simulink model "Invented_system_simulink_try"  (R2018b)
settings: Solver=VariableStepAuto  StartTime=0.0  StopTime=50  MaxStep=0.01  MinStep=0.00005  RelTol=1e-3
settings Model: Creator=ahmed  LastModifiedBy=ahmed

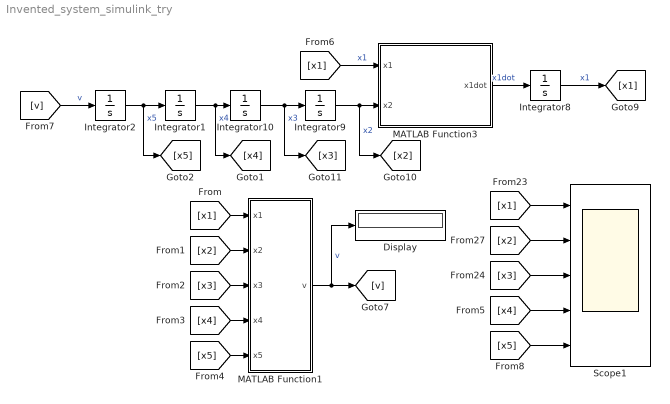
== system Invented_system_simulink_try ==
  Display : Display
      settings: Decimation=3
  Integrator1 : Integrator  InitialCondition=10
  Integrator10 : Integrator  InitialCondition=10
  Integrator2 : Integrator  InitialCondition=10
  Integrator8 : Integrator  InitialCondition=-10
  Integrator9 : Integrator  InitialCondition=20
  MATLAB Function1 : MATLAB Function  TreatAsAtomicUnit=on
  MATLAB Function3 : MATLAB Function  TreatAsAtomicUnit=on
  Scope1 : Scope  NumInputPorts=5
  wires:
  [x2] -> MATLAB Function1/2(x2)
  MATLAB Function1/1(v) -> Display/1, [v]  "v"
  [x1] -> Scope1/1
  [x1] -> MATLAB Function1/1(x1)
  [x3] -> MATLAB Function1/3(x3)
  MATLAB Function3/1(x1dot) -> Integrator8/1  "x1dot"
  Integrator8/1 -> [x1]  "x1"
  [x1] -> MATLAB Function3/1(x1)  "x1"
  Integrator9/1 -> [x2], MATLAB Function3/2(x2)  "x2"
  Integrator10/1 -> [x3], Integrator9/1  "x3"
  [v] -> Integrator2/1  "v"
  [x3] -> Scope1/3
  [x2] -> Scope1/2
  Integrator1/1 -> [x4], Integrator10/1  "x4"
  Integrator2/1 -> [x5], Integrator1/1  "x5"
  [x4] -> MATLAB Function1/4(x4)
  [x5] -> MATLAB Function1/5(x5)
  [x4] -> Scope1/4
  [x5] -> Scope1/5

== matlab function Invented_system_simulink_try/MATLAB Function1 ==
  data: x1 input; v output; x2 input; x3 input; x4 input; x5 input
function v = fcn(x1,x2,x3,x4,x5)

% Max step size 0.01
% Min step size auto
% not working initial conditions: x1=-10, x2=20, x3=10, x4=10, x5=10
% working initial conditions: x1=-10, x2=20, x3=-10, x4=10, x5=-10
% working initial conditions: x1=10, x2=20, x3=30, x4=40, x5=50
% working initial conditions: x1=1, x2=2, x3=3, x4=4, x5=5

% Max step size 0.01
% Min step size 0.00005
% all working

e2 = x2 + x1 + cos(x1);
e3 = x3 + 2*e2 - e2*sin(x1) + x1*sin(x1);

e4 = x4 + 3*e3 - e2 - 2*x1 - e3*sin(x1) + 2*e2*sin(x1) - e2^2*cos(x1) ...
    + 2*e2*x1*cos(x1) - x1^2*cos(x1);

e5 = x5 + 4*e4 - 3*e3 - 4*e2 + 3*x1 ...
   + e2^3*sin(x1) - x1^3*sin(x1) - e2*sin(x1) + 3*e3*sin(x1) - e4*sin(x1) ...
   - 2*x1*sin(x1) + 6*e2^2*cos(x1) - 3*e2*e3*cos(x1) - 6*e2*x1*cos(x1) ...
   + 3*e3*x1*cos(x1) + 3*e2*x1^2*sin(x1) - 3*e2^2*x1*sin(x1);

v = -5*e5 + 6*e4 + 5*e3 - 10*e2 - x1 ...
    + 12*e2^3*sin(x1) - 8*x1^2*cos(x1) - x1^4*cos(x1) + 4*e2*sin(x1) + 3*e3*sin(x1) ...
    - 4*e4*sin(x1) + e5*sin(x1) - 3*x1*sin(x1) + 16*e2^2*cos(x1) + 3*e3^2*cos(x1) ...
    - e2^4*cos(x1) - 24*e2*e3*cos(x1) + 4*e2*e4*cos(x1) + 4*e2*x1*cos(x1)...
    + 12*e3*x1*cos(x1) - 4*e4*x1*cos(x1) - 6*e2^2*e3*sin(x1) + 4*e2*x1^3*cos(x1) ...
    + 4*e2^3*x1*cos(x1) + 12*e2*x1^2*sin(x1) - 24*e2^2*x1*sin(x1) - 6*e3*x1^2*sin(x1) ...
    - 6*e2^2*x1^2*cos(x1) + 12*e2*e3*x1*sin(x1);

== matlab function Invented_system_simulink_try/MATLAB Function3 ==
  data: x1 input; x1dot output; x2 input
function x1dot = fcn(x1,x2)

x1dot = x2 + cos(x1);
